simulink library "MFMdl2"  (R2016b)
settings: Solver=VariableStepAuto  StartTime=0.0  StopTime=10.0  RelTol=1e-3
libraries: simulink x3
settings Model: Creator=viett  LastModifiedBy=viett

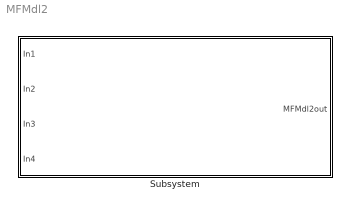
== system MFMdl2 ==
  Subsystem : Subsystem

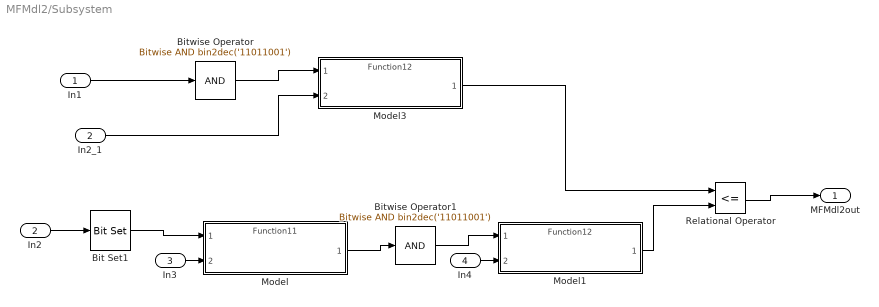
== system MFMdl2/Subsystem ==
  In1 : Inport
  In2 : Inport  Port=2
  In3 : Inport  Port=3
  In4 : Inport  Port=4
  Bit Set1 : simulink/Logic and Bit Operations/Bit Set  iBit=0
  Bitwise Operator : simulink/Logic and Bit Operations/Bitwise Operator  logicop=AND  UseBitMask=on  BitMask=bin2dec('11011001')  BitMaskRealWorld=Stored Integer
  Bitwise Operator1 : simulink/Logic and Bit Operations/Bitwise Operator  logicop=AND  UseBitMask=on  BitMask=bin2dec('11011001')  BitMaskRealWorld=Stored Integer
  In2_1 : InportShadow  Port=2
  Model : ModelReference  ModelNameDialog=Function11.slx  SimulationMode=Normal  ModelReferenceVersion=1.20
  Model1 : ModelReference  ModelNameDialog=Function12.slx  SimulationMode=Normal  ModelReferenceVersion=1.18
  Model3 : ModelReference  ModelNameDialog=Function12.slx  SimulationMode=Normal  ModelReferenceVersion=1.18
  Relational Operator : RelationalOperator  Operator=<=  OutDataTypeStr=boolean  RndMeth=Simplest
  MFMdl2out : Outport
  wires:
  In3/1 -> Model/2
  In2/1 -> Bit Set1/1
  In4/1 -> Model1/2
  Relational Operator/1 -> MFMdl2out/1
  Bit Set1/1 -> Model/1
  Model1/1 -> Relational Operator/2
  Model/1 -> Bitwise Operator1/1
  Bitwise Operator1/1 -> Model1/1
  Bitwise Operator/1 -> Model3/1
  Model3/1 -> Relational Operator/1
  In1/1 -> Bitwise Operator/1
  In2_1/1 -> Model3/2
